simulink subsystem "PvtSubSys_LATC"  (R2020b)
settings: Solver=VariableStepAuto  StartTime=0.0  StopTime=10.0  RelTol=1e-3
undefined symbols (not defined in the file or in its folder): P_Global_CharSpd_ms, P_Global_SteeringAngleRatio, P_Global_WheelBase_m, P_LCS_DetNoOverRide_DrvTrq_TH, P_LCS_DetOverRide_DrvTrq_TH, P_LCS_ESS_AngleSlope_Limit, P_LCS_ESS_LogicTest_Enable, P_LCS_ESS_NotActiveFlgDelayTime, P_LCS_ESS_NotActiveFlgDelayTimeSW, P_LCS_ESS_SteerAngleErr, P_LCS_ESS_SteerAngleFilterTime, P_LCS_ESS_TarAngleFilterTime, P_LCS_ESSAngleSW, P_LCS_ESSOverrideTime1, P_LCS_ESSOverrideTime2, P_LCS_ESSOverrideTime3, P_LCS_ESSOverrideValue1, P_LCS_ESSOverrideValue2, P_LCS_IN_Offset_Test_SW, P_LCS_IN_Offset_Test_Value, P_LCS_LATC_AngleFilterTime_s, P_LCS_LATC_CurOffsetCurve_TabX_m, P_LCS_LATC_CurOffsetCurveFliterTime_Tab_s, P_LCS_LATC_CurOffsetVehicleSpdLimitValue_degs, P_LCS_LATC_DeltaEps_Tab_s, P_LCS_LATC_DxOffset_Sw, P_LCS_LATC_ELKAngleSlope_ratio, P_LCS_LATC_ELKMaxLatAcc_ms2, P_LCS_LATC_ESSA0Dis_TabX_m, P_LCS_LATC_ESSAddAngleSlope_Tab_degs, P_LCS_LATC_ESSAESAngleSlope_Tab_degs, P_LCS_LATC_ESSAngleSlope_ratio, P_LCS_LATC_ESSMaxLatAcc_ms2, P_LCS_LATC_LCAngleSlope_ratio, P_LCS_LATC_LCAngleSlope_Tab_degs, P_LCS_LATC_LCCancleMaxLatAcc_ms2, P_LCS_LATC_LCEcoAngleSlope_ratio, P_LCS_LATC_LCEcoAngleSlope_Tab_degs, P_LCS_LATC_LCEcoMaxLatAcc_ms2, P_LCS_LATC_LCKAngleSlope_ratio, P_LCS_LATC_LCKAngleSlope_Tab_degs, P_LCS_LATC_LCKIEAngleSlope_ratio, P_LCS_LATC_LCKIEAngleSlope_Tab_degs, P_LCS_LATC_LCKIEMaxLatAcc_ms2, P_LCS_LATC_LCKMaxLatAcc_ms2, P_LCS_LATC_LCNormalAngleSlope_ratio, P_LCS_LATC_LCNormalAngleSlope_Tab_degs, P_LCS_LATC_LCNormalMaxLatAcc_ms2, P_LCS_LATC_LCSportAngleSlope_ratio, P_LCS_LATC_LCSportAngleSlope_Tab_degs, P_LCS_LATC_LCSportMaxLatAcc_ms2, P_LCS_LATC_LKAAngleSlope_ratio, P_LCS_LATC_LKAAngleSlope_Tab_degs, P_LCS_LATC_LKAMaxLatAcc_ms2, P_LCS_LATC_MatrixQ1_st, P_LCS_LATC_MatrixQ3_st, P_LCS_LATC_MatrixR_st, P_LCS_LATC_Preindex, P_LCS_LATC_PreWeight, P_LCS_LATC_StateActivAngleSlopeLimit_ratio ... (+64)
libraries: simulink x32
(part 4 of 5)

== system PvtSubSys_LATC/Subsystem/LateralControl/LCS_Angle/Motion_Planning/FrenetTrajectory/Subsystem/Switch Case Action Subsystem ==
  Flg : Inport
  StateHoldTime : Inport  Port=2
  Action Port : ActionPort
  ActiveAyDtLimit_TBL : Lookup_n-D  BreakpointsForDimension1=P_LCS_LATC_StateActiveFlg_TabX_st  BreakpointsForDimension2=P_LCS_LATC_StateActiveHoldTime_TabY_st  Table=P_LCS_PLAN_StateActiv_AyDtLimit_ms3  ExtrapMethod=Clip  UseLastTableValue=on  InternalRulePriority=Speed  OutDataTypeStr=single  RndMeth=Simplest
      settings: InputPortMap=u0,u1
  ActivePreviewT_TBL : Lookup_n-D  BreakpointsForDimension1=P_LCS_LATC_StateActiveFlg_TabX_st  BreakpointsForDimension2=P_LCS_LATC_StateActiveHoldTime_TabY_st  Table=P_LCS_PLAN_StateActiv_PreviewT_s  ExtrapMethod=Clip  UseLastTableValue=on  InternalRulePriority=Speed  OutDataTypeStr=single  RndMeth=Simplest
      settings: InputPortMap=u0,u1
  PreviewT : Outport
  AyDtLimit : Outport  Port=2
  wires:
  StateHoldTime/1 -> ActiveAyDtLimit_TBL/2, ActivePreviewT_TBL/2
  ActivePreviewT_TBL/1 -> PreviewT/1
  Flg/1 -> ActiveAyDtLimit_TBL/1, ActivePreviewT_TBL/1
  ActiveAyDtLimit_TBL/1 -> AyDtLimit/1

== system PvtSubSys_LATC/Subsystem/LateralControl/LCS_Angle/Motion_Planning/FrenetTrajectory/Subsystem/Switch Case Action Subsystem1 ==
  Action Port : ActionPort
  Constant : Constant  Value=100  OutDataTypeStr=single
  Constant1 : Constant  Value=100  OutDataTypeStr=single
  PreviewT : Outport
  AyDtLimit : Outport  Port=2
  wires:
  Constant/1 -> PreviewT/1
  Constant1/1 -> AyDtLimit/1

== system PvtSubSys_LATC/Subsystem/LateralControl/LCS_Angle/Motion_Planning/FrenetTrajectory_Lateral/Subsystem1/LP filter ==
  Raw : Inport
  TorqFilterTime : Inport  Port=2
  Product1 : Product  RndMeth=Zero
  Product4 : Product  Inputs=*/  RndMeth=Zero
  Sum4 : Sum  Inputs=+-
  Sum5 : Sum
  Unit Delay : UnitDelay  SampleTime=-1  HasFrameUpgradeWarning=on
  Weight/N3 : Constant  Value=0.02  OutDataTypeStr=single
  output : Outport
  wires:
  Sum5/1 -> output/1, Unit Delay/1
  Unit Delay/1 -> Sum5/2, Sum4/2
  Sum4/1 -> Product1/2
  Product1/1 -> Sum5/1
  Raw/1 -> Sum4/1
  Weight/N3/1 -> Product4/1
  Product4/1 -> Product1/1
  TorqFilterTime/1 -> Product4/2

== system PvtSubSys_LATC/Subsystem/LateralControl/LCS_Angle/Motion_Planning/FrenetTrajectory_Lateral/Subsystem1/Switch Case Action Subsystem ==
  Flg : Inport
  StateHoldTime : Inport  Port=2
  Action Port : ActionPort
  ActiveAyDtLimit_TBL : Lookup_n-D  BreakpointsForDimension1=P_LCS_LATC_StateActiveFlg_TabX_st  BreakpointsForDimension2=P_LCS_LATC_StateActiveHoldTime_TabY_st  Table=P_LCS_PLAN_StateActiv_AyDtLimit_ms3  ExtrapMethod=Clip  UseLastTableValue=on  InternalRulePriority=Speed  OutDataTypeStr=single  RndMeth=Simplest
      settings: InputPortMap=u0,u1
  ActivePreviewT_TBL : Lookup_n-D  BreakpointsForDimension1=P_LCS_LATC_StateActiveFlg_TabX_st  BreakpointsForDimension2=P_LCS_LATC_StateActiveHoldTime_TabY_st  Table=P_LCS_PLAN_StateActiv_PreviewT_s  ExtrapMethod=Clip  UseLastTableValue=on  InternalRulePriority=Speed  OutDataTypeStr=single  RndMeth=Simplest
      settings: InputPortMap=u0,u1
  PreviewT : Outport
  AyDtLimit : Outport  Port=2
  wires:
  StateHoldTime/1 -> ActiveAyDtLimit_TBL/2, ActivePreviewT_TBL/2
  ActivePreviewT_TBL/1 -> PreviewT/1
  Flg/1 -> ActiveAyDtLimit_TBL/1, ActivePreviewT_TBL/1
  ActiveAyDtLimit_TBL/1 -> AyDtLimit/1

== system PvtSubSys_LATC/Subsystem/LateralControl/LCS_Angle/Motion_Planning/FrenetTrajectory_Lateral/Subsystem1/Switch Case Action Subsystem1 ==
  Action Port : ActionPort
  Constant : Constant  Value=100  OutDataTypeStr=single
  Constant1 : Constant  Value=100  OutDataTypeStr=single
  PreviewT : Outport
  AyDtLimit : Outport  Port=2
  wires:
  Constant/1 -> PreviewT/1
  Constant1/1 -> AyDtLimit/1

== system PvtSubSys_LATC/Subsystem/LateralControl/LCS_Angle/Lateral_Control/MPC/TargetSteerAngleCalc/Subsystem/Switch Case Action Subsystem ==
  Flg : Inport
  StateHoldTime : Inport  Port=2
  Action Port : ActionPort
  LC_start_slope : Lookup_n-D  BreakpointsForDimension1=P_LCS_PLAN_StateActiveFlg_TabX_st  BreakpointsForDimension2=P_LCS_PLAN_StateActiveHoldTime_TabY_s  Table=P_LCS_PLAN_StateActivAngleSlope_Tab_ratio  ExtrapMethod=Clip  UseLastTableValue=on  InternalRulePriority=Speed  OutDataTypeStr=single  RndMeth=Simplest
      settings: InputPortMap=u0,u1
  Out1 : Outport
  wires:
  Flg/1 -> LC_start_slope/1
  LC_start_slope/1 -> Out1/1
  StateHoldTime/1 -> LC_start_slope/2

== system PvtSubSys_LATC/Subsystem/LateralControl/LCS_Angle/Lateral_Control/MPC/TargetSteerAngleCalc/Subsystem/Switch Case Action Subsystem1 ==
  Action Port : ActionPort
  Constant : Constant  Value=100  OutDataTypeStr=single
  Out1 : Outport
  wires:
  Constant/1 -> Out1/1

== system PvtSubSys_LATC/Subsystem/LateralControl/LCS_Angle/Lateral_Control/MPC/TargetSteerAngleCalc/Subsystem/Switch Case Action Subsystem2 ==
  Flg : Inport
  StateHoldTime : Inport  Port=2
  Action Port : ActionPort
  LC_start_slope : Lookup_n-D  BreakpointsForDimension1=P_LCS_PLAN_StateCompleteFlg_TabX_st  BreakpointsForDimension2=P_LCS_PLAN_StateActiveHoldTime_TabY_s  Table=P_LCS_PLAN_StateCompleteAngleSlope_Tab_ratio  ExtrapMethod=Clip  UseLastTableValue=on  InternalRulePriority=Speed  OutDataTypeStr=single  RndMeth=Simplest
      settings: InputPortMap=u0,u1
  Out1 : Outport
  wires:
  StateHoldTime/1 -> LC_start_slope/2
  LC_start_slope/1 -> Out1/1
  Flg/1 -> LC_start_slope/1

== system PvtSubSys_LATC/Subsystem/LateralControl/LCS_Angle/Lateral_Control/MPC/TargetSteerAngleCalc/Subsystem/Switch Case Action Subsystem3 ==
  Action Port : ActionPort
  Constant : Constant  Value=0.3  OutDataTypeStr=single
  Out1 : Outport
  wires:
  Constant/1 -> Out1/1

== system PvtSubSys_LATC/Subsystem/LateralControl/LCS_Angle/Lateral_Control/MPC/TargetSteerAngleCalc/Subsystem/Switch Case Action Subsystem4 ==
  Action Port : ActionPort
  Constant : Constant  OutDataTypeStr=single
  Out1 : Outport
  wires:
  Constant/1 -> Out1/1

== system PvtSubSys_LATC/Subsystem/LateralControl/LCS_Angle/Lateral_Control/MPC/TargetSteerAngleCalc/Subsystem/Switch Case Action Subsystem5 ==
  Flg : Inport
  StateHoldTime : Inport  Port=2
  Action Port : ActionPort
  LC_start_slope : Lookup_n-D  BreakpointsForDimension1=P_LCS_PLAN_StateCompleteFlg_TabX_st  BreakpointsForDimension2=P_LCS_PLAN_StateActiveHoldTime_TabY_s  Table=P_LCS_PLAN_LCCompletePreDisFac_Tab_ratio  ExtrapMethod=Clip  UseLastTableValue=on  InternalRulePriority=Speed  OutDataTypeStr=single  RndMeth=Simplest
      settings: InputPortMap=u0,u1
  LC_Complete_PreDisFac : Outport
  wires:
  Flg/1 -> LC_start_slope/1
  LC_start_slope/1 -> LC_Complete_PreDisFac/1
  StateHoldTime/1 -> LC_start_slope/2

== system PvtSubSys_LATC/Subsystem/LateralControl/LCS_Angle/Motion_Planning/CartesianTrajectory_MPC/Subsystem/Subsystem/Switch Case Action Subsystem ==
  Flg : Inport
  StateHoldTime : Inport  Port=2
  Action Port : ActionPort
  LC_start_slope : Lookup_n-D  BreakpointsForDimension1=P_LCS_PLAN_StateActiveFlg_TabX_st  BreakpointsForDimension2=P_LCS_PLAN_StateActiveHoldTime_TabY_s  Table=P_LCS_PLAN_StateActivAngleSlope_Tab_ratio  ExtrapMethod=Clip  UseLastTableValue=on  InternalRulePriority=Speed  OutDataTypeStr=single  RndMeth=Simplest
      settings: InputPortMap=u0,u1
  Out1 : Outport
  wires:
  Flg/1 -> LC_start_slope/1
  LC_start_slope/1 -> Out1/1
  StateHoldTime/1 -> LC_start_slope/2

== system PvtSubSys_LATC/Subsystem/LateralControl/LCS_Angle/Motion_Planning/CartesianTrajectory_MPC/Subsystem/Subsystem/Switch Case Action Subsystem1 ==
  Action Port : ActionPort
  Constant : Constant  Value=100  OutDataTypeStr=single
  Out1 : Outport
  wires:
  Constant/1 -> Out1/1

== system PvtSubSys_LATC/Subsystem/LateralControl/LCS_Angle/Motion_Planning/CartesianTrajectory_MPC/Subsystem/Subsystem/Switch Case Action Subsystem2 ==
  Flg : Inport
  StateHoldTime : Inport  Port=2
  Action Port : ActionPort
  LC_start_slope : Lookup_n-D  BreakpointsForDimension1=P_LCS_PLAN_StateCompleteFlg_TabX_st  BreakpointsForDimension2=P_LCS_PLAN_StateActiveHoldTime_TabY_s  Table=P_LCS_PLAN_StateCompleteAngleSlope_Tab_ratio  ExtrapMethod=Clip  UseLastTableValue=on  InternalRulePriority=Speed  OutDataTypeStr=single  RndMeth=Simplest
      settings: InputPortMap=u0,u1
  Out1 : Outport
  wires:
  StateHoldTime/1 -> LC_start_slope/2
  LC_start_slope/1 -> Out1/1
  Flg/1 -> LC_start_slope/1

== system PvtSubSys_LATC/Subsystem/LateralControl/LCS_Angle/Motion_Planning/CartesianTrajectory_MPC/Subsystem/Subsystem/Switch Case Action Subsystem3 ==
  Action Port : ActionPort
  Constant : Constant  Value=0.3  OutDataTypeStr=single
  Out1 : Outport
  wires:
  Constant/1 -> Out1/1

== system PvtSubSys_LATC/Subsystem/LateralControl/LCS_Angle/Motion_Planning/CartesianTrajectory_MPC/Subsystem/Subsystem/Switch Case Action Subsystem4 ==
  Action Port : ActionPort
  Constant : Constant  OutDataTypeStr=single
  Out1 : Outport
  wires:
  Constant/1 -> Out1/1

== system PvtSubSys_LATC/Subsystem/LateralControl/LCS_Angle/Motion_Planning/CartesianTrajectory_MPC/Subsystem/Subsystem/Switch Case Action Subsystem5 ==
  Flg : Inport
  StateHoldTime : Inport  Port=2
  Action Port : ActionPort
  LC_start_slope : Lookup_n-D  BreakpointsForDimension1=P_LCS_PLAN_StateCompleteFlg_TabX_st  BreakpointsForDimension2=P_LCS_PLAN_StateActiveHoldTime_TabY_s  Table=P_LCS_PLAN_LCCompletePreDisFac_Tab_ratio  ExtrapMethod=Clip  UseLastTableValue=on  InternalRulePriority=Speed  OutDataTypeStr=single  RndMeth=Simplest
      settings: InputPortMap=u0,u1
  LC_Complete_PreDisFac : Outport
  wires:
  Flg/1 -> LC_start_slope/1
  LC_start_slope/1 -> LC_Complete_PreDisFac/1
  StateHoldTime/1 -> LC_start_slope/2

== matlab function PvtSubSys_LATC/Subsystem/LateralControl/LCS_Angle/Motion_Planning/FrenetTrajectory_Lateral/FrenetTrajectory_Lateral ==
  data: A0 input; A1 input; A2 input; A3 input; Veh_Speed input size=1; YawRate input size=1; TarDangerlLevel input; PreView_T input size=1; PlanX output; PlanY output; PlanTheta output; idx output; PreviewX output; PreviewY output; PreviewTheta output; numTraj output size=1; ref_curvature output; AyDtLimit input size=1; Min_Plan_Dis input; lateral_error output size=1; lateral_error_rate output size=1; heading_error output size=1; heading_error_rate output size=1
function [PlanX,PlanY,PlanTheta,idx,PreviewX,PreviewY,PreviewTheta,numTraj,ref_curvature,lateral_error,lateral_error_rate,heading_error,heading_error_rate] ...
    = FrenetTrajectory_Lateral(A0,A1,A2,A3,Veh_Speed,YawRate,TarDangerlLevel,PreView_T,AyDtLimit,Min_Plan_Dis)
Veh_Speed = max(Veh_Speed,2);
%% 参考线离散化
rx1 = [single(0):single(1):single(19)];
rx2 = [single(20):20:150];
rx = cat(2,rx1,rx2);
ry = single((-1)).*(A0 + A1.* rx + A2.* (rx.^2) + A3.* (rx.^3));
waypoints = [ry',rx'];
referencePathPointNum = 100;
referencePath = FrenentReferencePath(waypoints,referencePathPointNum);
pathStart = referencePath.interpolate(0);% 求起始点处车辆状态 [x, y,theta, kappa, dkappa, s]
initialState=[0 -A0 pathStart(1,3)];

Frenet_traj_obj = TrajectoryGeneratorFrenet(referencePath);
FtNumTarpoints = single(40); % Frenet坐标系轨迹点数
GtNumTarpoints = single(40); % 全局坐标系轨迹点数
%% 生成轨迹
Py =single([1.5 2 2.5 3 3.6 4.4 5 5.8 6.4 7	7.8	8.6	9.5 10.4 11.4]);% 按等比1.1
Py = max(Veh_Speed,5) .* Py; % 暂时设定最短规划距离 5*2.5
Px = single((-1)).*(A3.*(Py.^3) + A2.*(Py.^2) + A1.*(Py.^1) + A0);
for i = 1:length(Py)
    arcLenOffsets = 1.05*sqrt(Px(i)^2 + Py(i)^2);
    [frenetTrajectory,globalTrajectory,numTraj] = Frenet_traj_obj.FrenetTrajectory_Lateral(initialState,arcLenOffsets,0,FtNumTarpoints,GtNumTarpoints);
    AyDt = (diff(frenetTrajectory.Trajectory(:,3).*(Veh_Speed*Veh_Speed)))./diff(frenetTrajectory.Trajectory(:,1)./Veh_Speed);
    if all(abs(AyDt(1:end,1)) < AyDtLimit) && (frenetTrajectory.Trajectory(end,1) > Min_Plan_Dis)
        break;
    end
end
numTraj = i;%借用numTraj将第几个时间点输出
[globalTrajectory] = EvaluateTrajectory_Lateral(frenetTrajectory,globalTrajectory, 1,1);
%%
% [s,d]→[x, y, theta, kappa, dkappa]
PlanX = single(zeros(GtNumTarpoints,1));
PlanY = single(zeros(GtNumTarpoints,1));
PlanTheta = single(zeros(GtNumTarpoints,1));
PlanX= globalTrajectory(1).Trajectory(1:GtNumTarpoints,2);
PlanY= globalTrajectory(1).Trajectory(1:GtNumTarpoints,1);
PlanTheta = globalTrajectory(1).Trajectory(1:GtNumTarpoints,3);
[matrix_state,ref_curvature,idx] = Calc_State_Error(Veh_Speed,YawRate,globalTrajectory,PreView_T,GtNumTarpoints);
PreviewX = globalTrajectory(1).Trajectory(idx,2);
PreviewY = globalTrajectory(1).Trajectory(idx,1);
PreviewTheta = globalTrajectory(1).Trajectory(idx,3);
% lateral_error = single(zeros(1,1));lateral_error_rate = single(zeros(1,1));heading_error = single(zeros(1,1));heading_error_rate = single(zeros(1,1));
lateral_error = matrix_state(1,1);
lateral_error_rate = matrix_state(2,1);
heading_error = matrix_state(3,1);
heading_error_rate = matrix_state(4,1);

end

== matlab function PvtSubSys_LATC/Subsystem/LateralControl/LCS_Angle/Motion_Planning/CartesianTrajectory_MPC/Subsystem/MATLAB Function3 ==
  data: delytime input uint16; TarDangerLevel input uint8; TarDangerLevelK1 input uint8; FLg output uint8; FLgK1 input uint8; CntK1 input uint16; Cnt output uint16
function [FLg,Cnt] = AngSlopeCalc(delytime,TarDangerLevel,TarDangerLevelK1,FLgK1,CntK1)

Cnt = min(CntK1 + uint16(1),delytime);
if Cnt== delytime
    FLg = uint8(0);
else
    FLg = FLgK1;
end
%FLg = FLgK1;
%% 换道开始检测
if TarDangerLevel==uint8(1) && TarDangerLevelK1==0  % NO function 2 LCK (TarDangerLevelK1==0)
    Cnt =uint16(0);
    FLg = uint8(1);
end
%由LCK状态切换为Normal
if  TarDangerLevel==uint8(3) && (TarDangerLevelK1==uint8(1)||TarDangerLevelK1==uint8(2)) % LCK/IE 2 LC_Normal
    Cnt =uint16(0);
    FLg = uint8(2);
end
%由LCK状态切换为Eco
if  TarDangerLevel==uint8(7) && (TarDangerLevelK1==uint8(1)||TarDangerLevelK1==uint8(2)) % LCK/IE 2 LC_Eco
    Cnt =uint16(0);
    FLg = uint8(3);
end
%由LCK状态切换为Sport
if  TarDangerLevel==uint8(8) && (TarDangerLevelK1==uint8(1)||TarDangerLevelK1==uint8(2)) % LCK/IE 2 LC_sport
    Cnt =uint16(0);
    FLg = uint8(4);
end
if  TarDangerLevel==uint8(6) && (TarDangerLevelK1==uint8(1)||TarDangerLevelK1==uint8(2)) % LCK/IE 2 ESS 后期添加配和ESS Slope 一起调试
    Cnt =uint16(0);
    FLg = uint8(5);
end
%% 换道完成检测，主要时为了解决换道完成后切换到LCK后Angleslope太小导致超调，检测到换道完成后延时一段时间保持一个大斜率。
if  (TarDangerLevel==uint8(1)||TarDangerLevel==uint8(2)) && (TarDangerLevelK1==uint8(3)) % LCK/IE 2 LC_Normal Complete
    Cnt =uint16(0);
    FLg = uint8(6);
end
if  (TarDangerLevel==uint8(1)||TarDangerLevel==uint8(2)) && (TarDangerLevelK1==uint8(7)) % LCK/IE 2 LC_Eco Complete
    Cnt =uint16(0);
    FLg = uint8(7);
end
if  (TarDangerLevel==uint8(1)||TarDangerLevel==uint8(2)) && (TarDangerLevelK1==uint8(8)) % LCK/IE 2 LC_sport Complete
    Cnt =uint16(0);
    FLg = uint8(8);
end

== matlab function PvtSubSys_LATC/Subsystem/LateralControl/LCS_Angle/Motion_Planning/FrenetTrajectory/FrenetTrajectory ==
  data: A0 input; A1 input; A2 input; A3 input; Veh_Speed input size=1; YawRate input size=1; PreView_T input size=1; PlanX output; PlanY output; PlanTheta output; idx output; PreviewX output; PreviewY output; PreviewTheta output; numTraj output size=1; ref_curvature output; AyDtLimit input size=1; Min_Plan_Dis input; lateral_error output size=1; lateral_error_rate output size=1; heading_error output size=1; heading_error_rate output size=1
function [PlanX,PlanY,PlanTheta,idx,PreviewX,PreviewY,PreviewTheta,numTraj,ref_curvature,lateral_error,lateral_error_rate,heading_error,heading_error_rate] ...
    = FrenetTrajectory(A0,A1,A2,A3,Veh_Speed,YawRate,PreView_T,AyDtLimit,Min_Plan_Dis)
% 参考线离散化
rx1 = [single(0):single(1):single(19)];
rx2 = [single(20):20:150];
rx = cat(2,rx1,rx2);   %将rx1 rx2两个横向量矩阵链接成一个新的行向量
ry = single((-1)).*(A0 + A1.* rx + A2.* (rx.^2) + A3.* (rx.^3));   %添加负号是将摄像头车道线转换为车体坐标
waypoints = [ry',rx'];
referencePathPointNum = 100; %参考轨迹的点的个数(参考点的分辨率)，此参数会影响最终目标轨迹线的形状，太小会出现轨迹线拐点
referencePath = FrenentReferencePath(waypoints,referencePathPointNum);   %通过路径点生成对应的平滑参考路径 
%FrenentReferencePath通过一组以[x y]或[x y θ]给出的路径点拟合出一个光滑的、分段的、连续的曲线。拟合后，沿曲线的点，路径点表示为[x y theta弧度 kappa曲率 dkappa曲率变化率 s弧长]，
%% 定义轨迹起始点状态
initGlobalState = [0 0 pi/2 0 Veh_Speed  0]; %暂时定义纵向加速度为0，[x, y,theta, kappa speed，Acc]  在全局坐标系下定义初始状态 我初始状态定义为 0         0    1.5708         0   45.0000         0
initFrenetState = referencePath.global2frenet(initGlobalState);  %在Frenet坐标系下定义初始状态  [S ds dds L dL ddL]  经过Frenet转换之后为0.0000   45.0000   -0.0092   -0.1200    0.0004         0   为什么横纵向会有一个加速度呢？  我给定的为一条近似的直线
% Py =single([2.5	2.7	3 3.3 3.6 4 4.4	4.8	5.3	5.8	6.4	7.1	7.8	8.6	9.5 10.4 11.4].*Py_Fac);
Py =single([1.5 2 2.5 3 3.6 4.2 5 5.8 6.4 7	7.8	8.6	9.5 10.4 11.4]);
TarEgoAy = zeros(1,length(Py));% 终点处期望纵向加速度
TarEgoV = ones(1,length(Py)) .* Veh_Speed;% 终点处期望纵向速度
Py = max(Veh_Speed,5).*Py;   %纵向行驶的距离
Px = single((-1)).*(A3.*(Py.^3) + A2.*(Py.^2) + A1.*(Py.^1) + A0);  %横向离参考线的距离

Frenet_traj_obj = TrajectoryGeneratorFrenet(referencePath);     %这个是干嘛的？   重新生成参考路径吗？？？？
FtNumTarpoints = single(40); % Frenet坐标系轨迹点数
%% 生成轨迹
for i = 1:length(Py)
    Pl = round(1.05*sqrt(Px(i)^2 + Py(i)^2));   
    Pt = round(1.05*sqrt(Px(i)^2 + Py(i)^2)/max(1,0.5*(TarEgoV(i) + Veh_Speed)));
    pathend= referencePath.interpolate(Pl);     %终点处对应路径点坐标[x y theta弧度 kappa曲率 dkappa曲率变化率 s弧长]
    EndGlobalState = [pathend(1:4) TarEgoV(i) TarEgoAy(i)];    %全局坐标下终了状态[x y theta弧度 kappa曲率 V a]
    EndFrenetState = referencePath.global2frenet(EndGlobalState);   %Frenet坐标系下终了状态[S ds dds L dL ddL]设定终了状态的横向距离 横向加速度 横向加加速度为零
    [frenetTrajectory,globalTrajectory] = Frenet_traj_obj.FrenetTrajectory(initFrenetState,EndFrenetState(1,1),0,EndFrenetState(1,2:3),EndFrenetState(1,5:6),Pt,FtNumTarpoints);
    AyDt = abs(diff(globalTrajectory.Trajectory(:,4).*((globalTrajectory.Trajectory(:,5).^2)))./diff(globalTrajectory.Times));
    if all(abs(AyDt)<AyDtLimit) && (frenetTrajectory.Trajectory(end,1) > Min_Plan_Dis)
        break;
    end
end
numTraj  = i;%借用numTraj输出时间点索引号
[globalTrajectory] = EvaluateTrajectory(frenetTrajectory,globalTrajectory,1,1,1,1);
%%
% [s,d]→[x, y, theta, kappa, dkappa]
PlanX = single(zeros(FtNumTarpoints,1));
PlanY = single(zeros(FtNumTarpoints,1));
PlanTheta = single(zeros(FtNumTarpoints,1));
PlanX= globalTrajectory(1).Trajectory(1:FtNumTarpoints,2);
PlanY= globalTrajectory(1).Trajectory(1:FtNumTarpoints,1);
PlanTheta = globalTrajectory(1).Trajectory(1:FtNumTarpoints,3);
[matrix_state,ref_curvature,idx] = Calc_State_Error(Veh_Speed,YawRate,globalTrajectory,PreView_T,FtNumTarpoints);
PreviewX = globalTrajectory(1).Trajectory(idx,2);
PreviewY = globalTrajectory(1).Trajectory(idx,1);
PreviewTheta = globalTrajectory(1).Trajectory(idx,3);
% lateral_error = single(zeros(1,1));lateral_error_rate = single(zeros(1,1));heading_error = single(zeros(1,1));heading_error_rate = single(zeros(1,1));
lateral_error = matrix_state(1,1);
lateral_error_rate = matrix_state(2,1);
heading_error = matrix_state(3,1);
heading_error_rate = matrix_state(4,1);

end

== stateflow chart PvtSubSys_LATC/Subsystem/LateralControl/LCS_Angle/OverRideDetect/Chart ==
  state NoOverRide
    en:isOverRide=false;
  state IsOverRide
    en:isOverRide=true;
  (default) -> NoOverRide
  NoOverRide -> IsOverRide : [Ovride]
  IsOverRide -> NoOverRide : [NoOvride]
  data: isOverRide output; Ovride input; NoOvride input

== matlab function PvtSubSys_LATC/Subsystem/LateralControl/LCS_Angle/Motion_Planning/FrenetTrajectory/Subsystem/MATLAB Function ==
  data: Forward_PreViewT input; VehSpd input; PreCurve output; C2 input; C3 input; PreCurve_Abs output
function [PreCurve,PreCurve_Abs]= PreView_Point_Curvature(Forward_PreViewT,VehSpd,C2,C3)
LookForwardDis = VehSpd * Forward_PreViewT;
PreCurve = 6*C3*LookForwardDis + 2*C2;
PreCurve_Abs = abs(PreCurve);
end

== matlab function PvtSubSys_LATC/Subsystem/LateralControl/LCS_Angle/Lateral_Control/MPC/TargetSteerAngleCalc/MATLAB Function3 ==
  data: delytime input uint16; TarDangerLevel input uint8; TarDangerLevelK1 input uint8; FLg output uint8; FLgK1 input uint8; CntK1 input uint16; Cnt output uint16
function [FLg,Cnt] = AngSlopeCalc(delytime,TarDangerLevel,TarDangerLevelK1,FLgK1,CntK1)

Cnt = min(CntK1 + uint16(1),delytime);
if Cnt== delytime
    FLg = uint8(0);
else
    FLg = FLgK1;
end
%FLg = FLgK1;
%% 换道开始检测
if TarDangerLevel==uint8(1) && TarDangerLevelK1==0  % NO function 2 LCK (TarDangerLevelK1==0)
    Cnt =uint16(0);
    FLg = uint8(1);
end
%由LCK状态切换为Normal
if  TarDangerLevel==uint8(3) && (TarDangerLevelK1==uint8(1)||TarDangerLevelK1==uint8(2)) % LCK/IE 2 LC_Normal
    Cnt =uint16(0);
    FLg = uint8(2);
end
%由LCK状态切换为Eco
if  TarDangerLevel==uint8(7) && (TarDangerLevelK1==uint8(1)||TarDangerLevelK1==uint8(2)) % LCK/IE 2 LC_Eco
    Cnt =uint16(0);
    FLg = uint8(3);
end
%由LCK状态切换为Sport
if  TarDangerLevel==uint8(8) && (TarDangerLevelK1==uint8(1)||TarDangerLevelK1==uint8(2)) % LCK/IE 2 LC_sport
    Cnt =uint16(0);
    FLg = uint8(4);
end
if  TarDangerLevel==uint8(6) && (TarDangerLevelK1==uint8(1)||TarDangerLevelK1==uint8(2)) % LCK/IE 2 ESS 后期添加配和ESS Slope 一起调试
    Cnt =uint16(0);
    FLg = uint8(5);
end
%% 换道完成检测，主要时为了解决换道完成后切换到LCK后Angleslope太小导致超调，检测到换道完成后延时一段时间保持一个大斜率。
if  (TarDangerLevel==uint8(1)||TarDangerLevel==uint8(2)) && (TarDangerLevelK1==uint8(3)) % LCK/IE 2 LC_Normal Complete
    Cnt =uint16(0);
    FLg = uint8(6);
end
if  (TarDangerLevel==uint8(1)||TarDangerLevel==uint8(2)) && (TarDangerLevelK1==uint8(7)) % LCK/IE 2 LC_Eco Complete
    Cnt =uint16(0);
    FLg = uint8(7);
end
if  (TarDangerLevel==uint8(1)||TarDangerLevel==uint8(2)) && (TarDangerLevelK1==uint8(8)) % LCK/IE 2 LC_sport Complete
    Cnt =uint16(0);
    FLg = uint8(8);
end

== matlab function PvtSubSys_LATC/Subsystem/LateralControl/LCS_Angle/Motion_Planning/CartesianTrajectory_MPC/CartesianTrajectory ==
  data: planX output single size=11; planY output single size=11; vEgo input size=1; planValid output boolean size=1; kapEgo input size=1; axEgo input size=1; TarLineValid input boolean size=1; TarLineC3 input size=1; TarLineC2 input size=1; TarLineC1 input size=1; TarLineC0 input size=1; ayDtLimit input size=1; planT output; LoopNum output; planLength output; Ay output size=11; AyDt output size=11; break_Flg output; break_AyValue output; break_AyDtValue output; PreDis input; Dis_Fac input; Min_PlanDis input
 function [planX,planY,planValid,planT,LoopNum,planLength,Ay,AyDt,break_Flg,break_AyValue,break_AyDtValue] = ...
    linePlanCalc(vEgo, kapEgo,axEgo,...
    TarLineValid,TarLineC3,TarLineC2,TarLineC1,TarLineC0,...
    ayDtLimit,PreDis,Dis_Fac,Min_PlanDis)
%五次多项式规划
LoopNum = 0;
if TarLineValid
    if (abs(TarLineC0)<single(0)) && (abs(TarLineC1)<single(0.05))  %控制线不走中心线，走规划线
        planValid = true;
        planT = single(11);
        planX = single(zeros(11,1));
        planY = single(zeros(11,1));
        planX = single((linspace(0,40,11)))';
        planY = TarLineC3.*planX.^3 + TarLineC2.*planX.^2 + TarLineC1*planX + TarLineC0;
        planLength = planX(end,1);
        Ay = single(zeros(11,1));
        AyDt = single(zeros(11,1));
        break_Flg = uint8(0);
        break_AyValue = single(0);
        break_AyDtValue = single(0);
    else
        Px =single([1.4 1.6 2.1 2.3 2.5 2.7 3 3.3 3.6 4 4.4 4.8 5.3 5.8 6.4 7.1 7.8 8.6 9.5 10.4 11.4]);% 按等比1.1  初选规划时间
        % 定义 TarEgoV、TarEgoAx，由于时间点数变化，导致轨迹条数变化，因此TarEgoV、TarEgoAx维数需要重新定义
        TarEgoAx = zeros(1,length(Px));
        TarEgoV = ones(1,length(Px)) .* vEgo;
        
        if vEgo>single(1)
            Px = vEgo*Px;   %纵向行驶距离
        end
        
        Py = TarLineC3*(Px.^3) + TarLineC2*(Px.^2) + TarLineC1*(Px.^1) + TarLineC0;
        x = single(zeros(11,1));
        y = single(zeros(11,1));
        Vx = single(zeros(11,1));
        Vy = single(zeros(11,1));
        Ax = single(zeros(11,1));
        Ay = single(zeros(11,1));
        AyDt = single(zeros(11,1));
        
        break_Flg = uint8(0);
        break_AyValue = single(0);
        break_AyDtValue = single(0);

        Pt = single(zeros(1,1));  
        for i = 1:length(Px)   
            Pt = 1.05*sqrt(Px(i)^2 + Py(i)^2)/max(1,0.5*(TarEgoV(i) + vEgo));  %规划时间
            t_Vego = max(vEgo,1);
            t0 = single(0);
            tn = Pt;
            
            T = [t0^5,t0^4,t0^3,t0^2,t0,1;...
                5*t0^4,4*t0^3,3*t0^2,2*t0,1,0;...
                20*t0^3,12*t0^2,6*t0,2,0,0;...
                tn^5,tn^4,tn^3,tn^2,tn,1;...
                5*tn^4,4*tn^3,3*tn^2,2*tn,1,0;...
                20*tn^3,12*tn^2,6*tn,2,0,0];    
            
            Vn = TarEgoV(i);
            An = TarEgoAx(i);
            kP =  3*TarLineC3*(Px(i).^2) + 2*TarLineC2*Px(i) + TarLineC1;  %规划线的斜率
            
            Kap = 6*TarLineC3*(Px(i))+2*TarLineC2;      
            Arcf = (vEgo^2)*Kap;                          
            Ayn = Arcf/sqrt(1 + kP^2);                       
            Axn = Arcf*kP/sqrt(1 + kP^2);                              
            Vxn = Vn/sqrt(1 + kP^2);                         
            Vyn = Vn*kP/sqrt(1 + kP^2);
            
            MaX = [0;t_Vego;axEgo;Px(i);Vxn;Axn];            
            MaY = [0;0;(vEgo^2)*kapEgo;Py(i);Vyn;Ayn];
            %求解多项式
            A = T\MaX;
            B = T\MaY;
            
            a5 = A(1);
            a4 = A(2);
            a3 = A(3);
            a2 = A(4);
            a1 = A(5);
            a0 = A(6);
            
            b5 = B(1);
            b4 = B(2);
            b3 = B(3);
            b2 = B(4);
            b1 = B(5);
            b0 = B(6);
            
            preLineValid = true;
            for j=1:11
                t = (j-1)*tn/10;
                x(j) = a5*t^5 + a4*t^4 + a3*t^3 + a2*t^2 + a1*t + a0;
                Vx(j) = 5*a5*t^4 + 4*a4*t^3 + 3*a3*t^2 + 2*a2*t + a1;
                Ax(j) = 20*a5*t^3 + 12*a4*t^2 + 6*a3*t + 2*a2;
                y(j) = b5*t^5 + b4*t^4 + b3*t^3 + b2*t^2 + b1*t + b0;
                Vy(j) = 5*b5*t^4 + 4*b4*t^3 + 3*b3*t^2 + 2*b2*t + b1;
                Ay(j) = 20*b5*t^3 + 12*b4*t^2 + 6*b3*t + 2*b2;
                AyDt(j) = 60*b5*t^2 + 24*b4*t + 6*b3;

                if (abs(AyDt(j))>ayDtLimit)
                    break_Flg = uint8(1);
                    break_AyValue = abs(Ay(j));
                    break_AyDtValue = abs(AyDt(j));
                    preLineValid = false;
                    break;
                end
            end
            if ((sqrt(x(11)^2 + y(11)^2)) < Min_PlanDis) || ((sqrt(x(11)^2 + y(11)^2))*Dis_Fac < (PreDis + 2.1))
                preLineValid = false;
            end
            if preLineValid
                break_Flg = uint8(3);
                break_AyValue = max(abs(Ay));
                break_AyDtValue = max(abs(AyDt(j)));
                break;
            end
            
            if i == length(Px) % 此处存在都不满足的情况，需要按最长时间输出。经测试发现如果按最长时间输出会控不住车辆。暂时改成跟随目标线
                planValid = true;
                Pt = single(Px(i));
                x = single(zeros(11,1));
                y = single(zeros(11,1));
                x = single((linspace(0,40,11)))';
                y = TarLineC3.*x.^3 + TarLineC2.*x.^2 + TarLineC1*x + TarLineC0;
                break_Flg = uint8(4);
                break_AyValue = single(0);
                break_AyDtValue = single(0);
            end
        end
        LoopNum = i;
        planValid = true;
        planT = Pt;
        planX = x;
        planY = y;
        planLength = planX(end,1);
    end
else
    planValid = false;
    planT = single(0);
    planX = single(zeros(11,1));
    planY = single(zeros(11,1));
    LoopNum = 0;
    planLength = planX(end,1);
    Ay = single(zeros(11,1));
    AyDt = single(zeros(11,1));
    break_Flg = uint8(0);
    break_AyValue = single(0);
    break_AyDtValue = single(0);
end

== matlab function PvtSubSys_LATC/Subsystem/LateralControl/LCS_Angle/Motion_Planning/FrenetTrajectory/Subsystem/MATLAB Function1 ==
  data: Delaytime input uint16; Flg output uint8; Count output uint16; TarDangerLevel input uint8; TarDangerLevelK1 input uint8; FlgK1 input uint8; CountK1 input uint16
function [Flg,Count]= fcn(Delaytime,TarDangerLevel,TarDangerLevelK1,FlgK1,CountK1)
Count = min(CountK1 + uint16(1),Delaytime);
if Count == Delaytime
    Flg = uint8(0);
else
    Flg = FlgK1;
end
%%状态检测
if TarDangerLevel == uint8(1) && TarDangerLevelK1 == 0 %功能激活
    Count = uint16(0);
    Flg = uint8(1);  
end
end

== matlab function PvtSubSys_LATC/Subsystem/LateralControl/EPSFaultCheck/MATLAB Function1 ==
  data: u input; y output uint8; countK input uint8; count output uint8
function [y,count] = fcn(u,countK)
count = countK - uint8(1);
if u>0
    count = uint8(3000);
end
if count > 1
    y = uint8(0);
else
    y = uint8(1);
end

== matlab function PvtSubSys_LATC/Subsystem/LateralControl/LCS_Angle/Lateral_Control/Dynamic_Model_LQR/TarSteerAngleCalc ==
  data: steer_angle_cmd_temp output; steer_feedforward_temp output; steer_feedbackward_temp output; steer_limit_temp output; LineValid input; SteerAngle input; steer_angle output size=[1,1]; Veh_Speed input; ref_curvature input; lateral_error input; lateral_error_rate input; heading_error input; heading_error_rate input; Left_steer_ratio input; Right_steer_ratio input; Matrix_q1 input; Matrix_q3 input; Matrix_R input; Max_lateral_acceleration input; TarSteerAngleSlope input; CurrentSteerAngleOffset input; steer_angleK1 input single
function [steer_angle_cmd_temp,steer_feedforward_temp,steer_feedbackward_temp,steer_limit_temp,steer_angle]= LQR_Algorithm(LineValid,SteerAngle,Veh_Speed,ref_curvature,lateral_error,lateral_error_rate,heading_error,heading_error_rate,...
    Left_steer_ratio,Right_steer_ratio,Matrix_q1,Matrix_q3,Matrix_R,Max_lateral_acceleration,TarSteerAngleSlope,CurrentSteerAngleOffset,steer_angleK1)
if LineValid
    %% 1.车辆参数
    %1.1 车的大小及长度参数
    veh_params.vehicle_length = single(4.875);
    veh_params.vehicle_width  = single(2.2);
    veh_params.vehicle_height = single(1.69);
    %1.2 车辆控制参数
    veh_params.wheel_base = single(2.92);               %轴距, m
    veh_params.Vch = single(23.5);                      %特征车速
    veh_params.max_steer_angle = single(53 / 180 * pi); %前轮最大转角
    veh_params.max_acceleration = single(2);            %车辆最大加速度
    veh_params.max_deceleration = single(-2);           %车辆最大减速度
    veh_params.left_steer_ratio = Left_steer_ratio;     %车辆左侧转向传动比%
    veh_params.right_steer_ratio = Right_steer_ratio;   %车辆右侧转向传动比%
    veh_params.cf = single(155494.663);                 %车辆前轮侧偏刚度
    veh_params.cr = single(155494.663);                 %车辆后轮侧偏刚度 
    veh_params.mass_fl = single(520);                   %车辆左前轮负重
    veh_params.mass_fr = single(520);                   %车辆右前轮负重
    veh_params.mass_rl = single(520);                   %车辆左后轮负重
    veh_params.mass_rr = single(520);                   %车辆右后轮负重
    %% 2.控制参数计算
    mass_front =  veh_params.mass_fl + veh_params.mass_fr;      %前轮负载
    mass_rear  =  veh_params.mass_rl + veh_params.mass_rr;      %后轮负载
    mass =  mass_front + mass_rear;                             %整车负载
    lf = veh_params.wheel_base * (single(1.0) - mass_front / mass);  %质心到前轴的距离
    lr = veh_params.wheel_base * (single(1.0) - mass_rear / mass);   %质心到后轴的距离
    iz = lf * lf * mass_front + lr * lr * mass_rear;                 %整车绕Z轴转动惯量
    %% 3.LQR参数设置
    
    lqr_eps = single(0.01);
    lqr_max_iteration = single(800);
    
    basic_state_size = uint8(4);
    control_size = uint8(1);
    
    matrix_a = single(zeros(basic_state_size,basic_state_size));           %定义状态方程A矩阵 4*4
    matrix_a_coeff = single(zeros(basic_state_size,basic_state_size));
    I = single(eye(basic_state_size,basic_state_size));                    %定义I为4*4的单位矩阵     这个矩阵是干嘛的？
    matrix_a(1,2) = single(1.0);
    matrix_a(2,3) = single((veh_params.cf + veh_params.cr ) / mass);
    matrix_a(3,4) = single(1.0);
    matrix_a(4,3) = single((lf * veh_params.cf - lr * veh_params.cr) / iz);
    
    matrix_a_coeff(2,2) = single(-(veh_params.cf + veh_params.cr) / mass);
    matrix_a_coeff(2,4) = single((lr * veh_params.cr - lf * veh_params.cf) / mass);
    matrix_a_coeff(3,4) = single(1.0);
    matrix_a_coeff(4,2) = single((lr * veh_params.cr - lf * veh_params.cf) / iz);
    matrix_a_coeff(4,4) = single(-1.0 * (lf * lf * veh_params.cf + lr * lr * veh_params.cr)/iz);
    
    matrix_a(2,2) = matrix_a_coeff(2,2);
    matrix_a(2,4) = matrix_a_coeff(2,4);
    matrix_a(4,2) = matrix_a_coeff(4,2);
    matrix_a(4,4) = matrix_a_coeff(4,4);
    
    matrix_b = single(zeros(basic_state_size,control_size));               %定义状态方程B矩阵 4*1
    matrix_b(2,1) = veh_params.cf/mass;
    matrix_b(4,1) = lf * veh_params.cf /iz;
    
    matrix_q = single(zeros(4,4));                  %定义Q矩阵为4*4零矩阵   理论应该定义Q矩阵为4*4的单位阵  此处这样定义忽略了横向误差率以及航向误差率
    matrix_q(1,1) = Matrix_q1;                      %调整q矩阵的第一、三个参数，改善转向性能0.0001,0.02  Q为状态权重系数
    matrix_q(3,3) = Matrix_q3;
    matrix_r = single(zeros(1,1));                  %定义R矩阵
    matrix_r = Matrix_R;                            %R为控制量权重系数
    
    lqr_params.A = matrix_a;
    lqr_params.B = matrix_b;
    lqr_params.I = I;
    lqr_params.ts = single(0.02);                  %预测时间
    lqr_params.lr = lr;
    lqr_params.lf = lf;
    lqr_params.cf=veh_params.cf;
    lqr_params.cr=veh_params.cr;
    lqr_params.iz=iz;                              %转动惯量
    lqr_params.mass=mass;
    lqr_params.Q =matrix_q ;
    lqr_params.R = matrix_r;
    lqr_params.eps=lqr_eps;
    lqr_params.max_iteration=lqr_max_iteration;
    %% 4.计算前轮转角
    lqr_params.A(2,2) = lqr_params.A(2,2)/(max(Veh_Speed, single(0.2)));
    lqr_params.A(2,4) = lqr_params.A(2,4)/(max(Veh_Speed, single(0.2)));
    lqr_params.A(4,2) = lqr_params.A(4,2)/(max(Veh_Speed, single(0.2)));
    lqr_params.A(4,4) = lqr_params.A(4,4)/(max(Veh_Speed, single(0.2)));
    
    A=lqr_params.A;
    B=lqr_params.B;
    I=lqr_params.I;
    ts=lqr_params.ts;      %控制周期
    min_tol = lqr_params.eps;    %0.01  这个时间是什么意思？？？？？？
    max_iter = lqr_params.max_iteration;   %800   这个是什么意思？？？？？
    matrix_Q = lqr_params.Q;
    matrix_R = lqr_params.R;
    
    matrix_ad=single(zeros(size(A)));   %4*4零矩阵
    matrix_ad=(I+ts*single(0.5) * A) / (I-ts*single(0.5) * A);  %控制是一个离散系统，而状态方程是一个连续的系统 因此需要离散 运用双线性离散化的方法离散
    
    matrix_bd=single(zeros(size(B)));
    matrix_bd=B*ts;
    matrix_k = SolveLQRProblem(matrix_ad, matrix_bd, matrix_Q,matrix_R, min_tol, max_iter);  %求解最优解K
    %% 横向控制状态变量
    
    matrix_state = single(zeros(4, 1));
    matrix_state(1, 1) = lateral_error;                   %横向误差
    matrix_state(2, 1) = lateral_error_rate;              %横向误差率
    matrix_state(3, 1) = heading_error;                   %航向误差
    matrix_state(4, 1) = heading_error_rate;              %航向误差率
    steer_feedbackward = -(matrix_k * matrix_state);      %-Kx   反馈
    % 计算前馈转向角
    kv = lqr_params.lr * lqr_params.mass / single(1) / lqr_params.cf / veh_params.wheel_base - ...
        lqr_params.lf * lqr_params.mass / single(1) / lqr_params.cr / veh_params.wheel_base;       %不足转向斜率
    steer_feedforward = (veh_params.wheel_base * ref_curvature + kv * Veh_Speed * Veh_Speed * ref_curvature - matrix_k(1, 3) * ...
        (lqr_params.lr * ref_curvature - lqr_params.lf * lqr_params.mass * Veh_Speed * Veh_Speed * ref_curvature / single(1) / lqr_params.cr / veh_params.wheel_base));%弧度制角度rad
    % 4.3 计算期望前轮偏角
    steer_cmd = steer_feedforward + steer_feedbackward;
    
    if (steer_cmd>=0)
        steer_transmission_ratio = veh_params.left_steer_ratio;
    else
        steer_transmission_ratio = veh_params.right_steer_ratio;
    end
    steer_feedforward_temp = steer_feedforward * single(57.3) * steer_transmission_ratio;%前馈计算的方向盘转角
    steer_feedbackward_temp = steer_feedbackward * single(57.3) * steer_transmission_ratio;%反馈计算的方向盘转角
    steer_angle_cmd = steer_cmd * single(57.3) * steer_transmission_ratio;%期望方向盘转角
    steer_angle_cmd_temp = steer_angle_cmd;%输出算法计算角度作为观测，最终请求角度会补偿转向不足。  角度值
    %% 5.限制期望前轮偏角
    % 5.1 根据横向加速度限制前轮转角
    if Veh_Speed < 1
        steer_limit = atan( Max_lateral_acceleration * veh_params.wheel_base /(Veh_Speed *Veh_Speed))* single(57.3) * steer_transmission_ratio; % 高速计算不准确，更改为下面特征车速计算方法
    else
        AckConst = min((single(1)+Veh_Speed*Veh_Speed/(veh_params.Vch*veh_params.Vch))*veh_params.wheel_base/max(single(1),Veh_Speed),single(32767));      %单位s2
        % PsiDtAckRaw = (SteerAngle/steer_transmission_ratio)/AckConst;
        steer_limit = ((Max_lateral_acceleration * AckConst)/Veh_Speed)* single(57.3) * steer_transmission_ratio;    %弧度转换为°  
    end
    %     steer_limit = atan( Max_lateral_acceleration * veh_params.wheel_base /(Veh_Speed *Veh_Speed)) * steer_transmission_ratio;
    steer_angle_cmd = min(steer_limit, max(-steer_limit,steer_angle_cmd));%前轮限制转角
    
    steer_angle_deg = steer_angle_cmd + CurrentSteerAngleOffset;      %最终输出的方向盘转角    
    steer_limit_temp = steer_limit;
    % 5.2 限制方向盘转速
    steer_angle = min(steer_angleK1 + TarSteerAngleSlope,max(steer_angleK1 - TarSteerAngleSlope,steer_angle_deg));
    
else
    steer_angle = SteerAngle;
    steer_angle_cmd_temp = single(0);
    steer_feedforward_temp = single(0);
    steer_feedbackward_temp = single(0);
    steer_limit_temp = single(0);
end
end

== matlab function PvtSubSys_LATC/Subsystem/LateralControl/LCS_Angle/Motion_Planning/CartesianTrajectory/Subsystem1/MATLAB Function ==
  data: Forward_PreViewT input; VehSpd input; PreCurve output; C2 input; C3 input; PreCurve_Abs output
function [PreCurve,PreCurve_Abs]= PreView_Point_Curvature(Forward_PreViewT,VehSpd,C2,C3)
LookForwardDis = VehSpd * Forward_PreViewT;
PreCurve = 6*C3*LookForwardDis + 2*C2;
PreCurve_Abs = abs(PreCurve);
end

== matlab function PvtSubSys_LATC/Subsystem/LateralControl/LCS_Angle/Motion_Planning/CartesianTrajectory/Subsystem1/MATLAB Function1 ==
  data: Delaytime input uint16; Flg output uint8; Count output uint16; TarDangerLevel input uint8; TarDangerLevelK1 input uint8; FlgK1 input uint8; CountK1 input uint16
function [Flg,Count]= fcn(Delaytime,TarDangerLevel,TarDangerLevelK1,FlgK1,CountK1)
Count = min(CountK1 + uint16(1),Delaytime);
if Count == Delaytime
    Flg = uint8(0);
else
    Flg = FlgK1;
end
%%状态检测
if TarDangerLevel == uint8(1) && TarDangerLevelK1 == 0 %功能激活
    Count = uint16(0);
    Flg = uint8(1);  
end
end

== matlab function PvtSubSys_LATC/Subsystem/LateralControl/LCS_Angle/Motion_Planning/CartesianTrajectory/FrenetTrajectory ==
  data: A0 input; A1 input; A2 input; A3 input; Veh_Speed input size=1; YawRate input size=1; PreView_T input size=1; PlanX output; PlanY output; PlanTheta output; idx output; PreviewX output; PreviewY output; PreviewTheta output; numTraj output size=1; ref_curvature output; AyDtLimit input size=1; Min_Plan_Dis input; lateral_error output size=1; lateral_error_rate output size=1; heading_error output size=1; heading_error_rate output size=1; axEgo input; kapEgo input
function [PlanX,PlanY,PlanTheta,idx,PreviewX,PreviewY,PreviewTheta,numTraj,ref_curvature,lateral_error,lateral_error_rate,heading_error,heading_error_rate] ...
    = FrenetTrajectory(A0,A1,A2,A3,Veh_Speed,YawRate,PreView_T,AyDtLimit,Min_Plan_Dis,axEgo,kapEgo)
%% 生成轨迹
Px =single([1.5 2 2.5 2.7 3 3.3 3.6 4 4.4 4.8 5.3 5.8 6.4 7.1 7.8 8.6 9.5 10.4 11.4]); %Py_Fac后期去掉，增加一个轨迹筛选条件，每个车速下最小规划距离
TarEgoAx = zeros(1,length(Px));   %初始化矩阵
TarEgoV = ones(1,length(Px)) .* Veh_Speed;  %计算纵向行驶距离
if Veh_Speed>single(1)
    Px = Veh_Speed*Px;    %纵向距离 l 
end 
Py = A3*(Px.^3) + A2*(Px.^2) + A1*(Px.^1) + A0;  
x = single(zeros(11,1));
y = single(zeros(11,1));
Vx = single(zeros(11,1));
Vy = single(zeros(11,1));
Ax = single(zeros(11,1));
Ay = single(zeros(11,1));
AyDt = single(zeros(11,1));
Pt = single(zeros(1,1));
for i = 1:length(Py)
    Pt = 1.05*sqrt(Px(i)^2 + Py(i)^2)/max(1,0.5*(TarEgoV(i) + Veh_Speed));
    t_Vego = max(Veh_Speed,1);
    t0 = single(0);
    tn = Pt;
    T = [t0^5,t0^4,t0^3,t0^2,t0,1;...
        5*t0^4,4*t0^3,3*t0^2,2*t0,1,0;...
        20*t0^3,12*t0^2,6*t0,2,0,0;...
        tn^5,tn^4,tn^3,tn^2,tn,1;...
        5*tn^4,4*tn^3,3*tn^2,2*tn,1,0;...
        20*tn^3,12*tn^2,6*tn,2,0,0];
    Vn = TarEgoV(i);
    An = TarEgoAx(i);
    kP =  3*A3*(Px(i).^2) + 2*A2*Px(i) + A1;
    
    Kap = 6*A3*(Px(i))+2*A2;
    Arcf = (Veh_Speed^2)*Kap;
    Ayn = Arcf/sqrt(1 + kP^2);
    Axn = Arcf*kP/sqrt(1 + kP^2);
    
    Vxn = Vn/sqrt(1 + kP^2);
    Vyn = Vn*kP/sqrt(1 + kP^2);
    MaX = [0;t_Vego;axEgo;Px(i);Vxn;Axn];
    MaY = [0;0;(Veh_Speed^2)*kapEgo;Py(i);Vyn;Ayn];
    A = T\MaX;
    B = T\MaY;
    
    a5 = A(1); % 纵向轨迹系数
    a4 = A(2);
    a3 = A(3);
    a2 = A(4);
    a1 = A(5);
    a0 = A(6);
    
    b5 = B(1); % 横向轨迹系数
    b4 = B(2);
    b3 = B(3);
    b2 = B(4);
    b1 = B(5);
    b0 = B(6);
    preLineValid = true;
    for j=1:11
        t = (j-1)*tn/10;
        x(j) = a5*t^5 + a4*t^4 + a3*t^3 + a2*t^2 + a1*t + a0;
        Vx(j) = 5*a5*t^4 + 4*a4*t^3 + 3*a3*t^2 + 2*a2*t + a1;
        Ax(j) = 20*a5*t^3 + 12*a4*t^2 + 6*a3*t + 2*a2;
        y(j) = b5*t^5 + b4*t^4 + b3*t^3 + b2*t^2 + b1*t + b0;
        Vy(j) = 5*b5*t^4 + 4*b4*t^3 + 3*b3*t^2 + 2*b2*t + b1;
        Ay(j) = 20*b5*t^3 + 12*b4*t^2 + 6*b3*t + 2*b2;
        AyDt(j) = 60*b5*t^2 + 24*b4*t + 6*b3;
        if abs(AyDt(j))>AyDtLimit 
            preLineValid = false;
            break;
        end     
    end
    if abs(sqrt(x(11)^2+y(11)^2)) < Min_Plan_Dis
       preLineValid = false; 
    end
    if preLineValid
        break;
    end
end
NumTarpoints = 40;
y = y.*single(-1);
objSpline = Spline2D(y,x);
s = single(linspace(0,objSpline.s(end),NumTarpoints));
TargetPoints = single(zeros(length(s),6));
for i = single(1):single(1):length(s)
    [ix,iy] = objSpline.calc_position(s(i));
    TargetPoints(i,1) = ix;
    TargetPoints(i,2) = iy;
    TargetPoints(i,3) = objSpline.calc_yaw(s(i));
    TargetPoints(i,4) = objSpline.calc_curvature(s(i));
    TargetPoints(i,5) = objSpline.calc_curvatureDerivative(s(i));
    TargetPoints(i,6) = s(i);
end
traj = single(zeros(NumTarpoints,6)); t= single(zeros(NumTarpoints,1)); costs = single(zeros(1,1));
globalTrajectory = repmat(struct('Trajectory',traj,'Times',t,'costs',costs), 1, 1);
globalTrajectory(1).Trajectory = TargetPoints;
globalTrajectory(1).Times = t;

numTraj  = i;%借用numTraj输出时间点索引号
%%
% [s,d]→[x, y, theta, kappa, dkappa]
PlanX= globalTrajectory(1).Trajectory(1:NumTarpoints,2);
PlanY= globalTrajectory(1).Trajectory(1:NumTarpoints,1);
PlanTheta = globalTrajectory(1).Trajectory(1:NumTarpoints,3);
[matrix_state,ref_curvature,idx] = Calc_State_Error(Veh_Speed,YawRate,globalTrajectory,PreView_T,NumTarpoints);
PreviewX = globalTrajectory(1).Trajectory(idx,2);
PreviewY = globalTrajectory(1).Trajectory(idx,1);
PreviewTheta = globalTrajectory(1).Trajectory(idx,3);
% lateral_error = single(zeros(1,1));lateral_error_rate = single(zeros(1,1));heading_error = single(zeros(1,1));heading_error_rate = single(zeros(1,1));
lateral_error = matrix_state(1,1);
lateral_error_rate = matrix_state(2,1);
heading_error = matrix_state(3,1);
heading_error_rate = matrix_state(4,1);

end

== matlab function PvtSubSys_LATC/Subsystem/LateralControl/ESS_SteerSpd_Test/NotActiveFlgDelayTime/MATLAB Function ==
  data: FlgIn input boolean; FlgOut output boolean size=1; t_offset input single; tcycle input single; FlgOutK1 input boolean; delaytimeK1 input single; delaytime output single size=1; flgK1 input uint8; flg output uint8 size=1
function [FlgOut,delaytime,flg]= fcn(FlgIn,t_offset,tcycle,FlgOutK1,delaytimeK1,flgK1)
FlgOut = FlgIn;
delaytime = single(0);
flg = uint8(0);
if FlgOutK1 ==0 && FlgOut == 1
    flg = uint8(1);
    FlgOut = true;
    delaytime = tcycle;
end
if  flgK1 == 1
     delaytime = delaytimeK1 + tcycle;
      if delaytime < t_offset
          flg = uint8(1);
          FlgOut = true;
      end
end

== matlab function PvtSubSys_LATC/Subsystem/LateralControl/LCS_Angle/Lateral_Control/MPC/Understeer&Offset_Calc/YOD_Ackman ==
  data: AckConst output; VxvRef input; Vch input; WheelBase input; AlpWheelAngle input; PsiDtAckK1 input single; PsiDtAck output
function [AckConst,PsiDtAck] = Ackman(VxvRef,Vch,WheelBase,AlpWheelAngle,PsiDtAckK1)
%#codegen
if VxvRef==uint8(0)%转换常数数据类型
    PsiDtAckRaw = single(0);%转换常数数据类型
    AckConst = single(1);%转换常数数据类型
else
    AckConst = min((single(1)+VxvRef*VxvRef/(Vch*Vch))*WheelBase/VxvRef,single(32767));%转换常数数据类型
    PsiDtAckRaw = AlpWheelAngle/AckConst;
end
PsiDtAck = (single(0.02/0.1))*(PsiDtAckRaw-PsiDtAckK1)+PsiDtAckK1;%转换常数数据类型

== matlab function PvtSubSys_LATC/Subsystem/LateralControl/LCS_Angle/Motion_Planning/FrenetTrajectory_Lateral/Subsystem1/MATLAB Function ==
  data: Forward_PreViewT input; VehSpd input; PreCurve output; C2 input; C3 input; PreCurve_Abs output
function [PreCurve,PreCurve_Abs]= PreView_Point_Curvature(Forward_PreViewT,VehSpd,C2,C3)
LookForwardDis = VehSpd * Forward_PreViewT;
PreCurve = 6*C3*LookForwardDis + 2*C2;
PreCurve_Abs = abs(PreCurve);
end

== matlab function PvtSubSys_LATC/Subsystem/LateralControl/LCS_Angle/Lateral_Control/MPC/TargetSteerAngleCalc/MATLAB Function ==
  data: c2 input; c1 input; c3 input; v input; PreCurve output; time input
function PreCurve = fcn(c2,c1,c3,v,time)
pdis = v*time;
% y1 = 3*c3*pdis^2 + 2*c2*pdis + c1;
PreCurve = 6*c3*pdis + 2*c2;
% r = y2/power((1+y1*y1),single(1.5));
end

== matlab function PvtSubSys_LATC/Subsystem/LateralControl/LCS_Angle/Motion_Planning/FrenetTrajectory_Lateral/Subsystem1/MATLAB Function1 ==
  data: Delaytime input uint16; Flg output uint8; Count output uint16; TarDangerLevel input uint8; TarDangerLevelK1 input uint8; FlgK1 input uint8; CountK1 input uint16
function [Flg,Count]= fcn(Delaytime,TarDangerLevel,TarDangerLevelK1,FlgK1,CountK1)
Count = min(CountK1 + uint16(1),Delaytime);
if Count == Delaytime
    Flg = uint8(0);
else
    Flg = FlgK1;
end
%%状态检测
if TarDangerLevel == uint8(1) && TarDangerLevelK1 == 0 %功能激活
    Count = uint16(0);
    Flg = uint8(1);  
end
end

== matlab function PvtSubSys_LATC/Subsystem/LateralControl/LCS_Angle/Motion_Planning/CartesianTrajectory_MPC/Subsystem/MATLAB Function ==
  data: c2 input; c1 input; c3 input; v input; PreCurve output; time input
function PreCurve = fcn(c2,c1,c3,v,time)
pdis = v*time;
% y1 = 3*c3*pdis^2 + 2*c2*pdis + c1;
PreCurve = 6*c3*pdis + 2*c2;
% r = y2/power((1+y1*y1),single(1.5));
end
